simulink model "SmallSupplyChain"  (Simulink 7.9)
settings: Solver=VariableStepDiscrete  StartTime=0.0  StopTime=1000.0  RelTol=1e-3
undefined symbols (not defined in the file): des, gcbh
libraries: se_batching x2
settings Model: Creator=tsprock3  LastModifiedBy=tsprock3
settings DebuggingCC: SimStateOlderReleaseMsg=warning

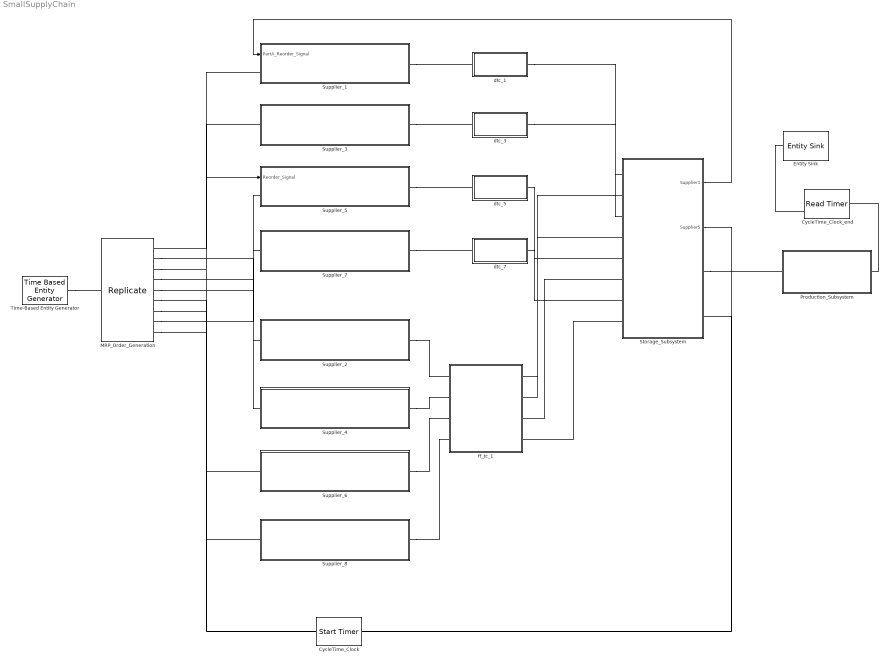
== system SmallSupplyChain ==
  CycleTime_Clock : StartTimer
  CycleTime_Clock_end : ReadTimer  TimerModeOption=Ignore  StatAverageTimeElapsed=on
      settings: OutputPortMap=o3
  Entity Sink : EntitySink
  MRP_Order_Generation : Replicate  NumberOutputPorts=9  ReplicateEntityWhen=Any entity output port is not blocked
  Production_Subsystem : Subsystem  TreatAsAtomicUnit=on
  Storage_Subsystem : Subsystem  TreatAsAtomicUnit=on
  Supplier_1 : Subsystem
  Supplier_2 : Subsystem
  Supplier_3 : Subsystem
  Supplier_4 : Subsystem
  Supplier_5 : Subsystem  mask{NumberOfServers=1, Capacity=25}
      mask prompts: NumberOfServers "Number of servers:"
  Supplier_6 : Subsystem
  Supplier_7 : Subsystem
  Supplier_8 : Subsystem
  Time-Based Entity Generator : TimeBasedEntityGenerator  Period=5
  dtc_1 : Subsystem
  dtc_3 : Subsystem
  dtc_5 : Subsystem
  dtc_7 : Subsystem
  ff_tc_1 : Subsystem  TreatAsAtomicUnit=on
  wires:
  Storage_Subsystem/1(Supplier1) -> Supplier_1/1(PartA_Reorder_Signal)
  Storage_Subsystem/2(Supplier5) -> Supplier_5/1(Reorder_Signal)
  connections:
  MRP_Order_Generation/RConn2 -- Supplier_2/LConn1
  MRP_Order_Generation/RConn4 -- Supplier_4/LConn1
  MRP_Order_Generation/RConn6 -- Supplier_6/LConn1
  MRP_Order_Generation/RConn8 -- Supplier_7/LConn1
  MRP_Order_Generation/RConn7 -- Supplier_8/LConn1
  Supplier_1/RConn1 -- dtc_1/LConn1
  Supplier_3/RConn1 -- dtc_3/LConn1
  Supplier_5/RConn1 -- dtc_5/LConn1
  Supplier_7/RConn1 -- dtc_7/LConn1
  Storage_Subsystem/RConn1 -- Production_Subsystem/LConn1
  dtc_1/RConn1 -- Storage_Subsystem/LConn1
  dtc_3/RConn1 -- Storage_Subsystem/LConn3
  dtc_5/RConn1 -- Storage_Subsystem/LConn5
  dtc_7/RConn1 -- Storage_Subsystem/LConn7
  Time-Based Entity Generator/RConn1 -- MRP_Order_Generation/LConn1
  Production_Subsystem/RConn1 -- CycleTime_Clock_end/LConn1
  CycleTime_Clock_end/RConn1 -- Entity Sink/LConn1
  MRP_Order_Generation/RConn9 -- CycleTime_Clock/LConn1
  CycleTime_Clock/RConn1 -- Storage_Subsystem/RConn2
  Supplier_1/LConn1 -- MRP_Order_Generation/RConn1
  MRP_Order_Generation/RConn3 -- Supplier_3/LConn1
  MRP_Order_Generation/RConn5 -- Supplier_5/LConn1
  Supplier_2/RConn1 -- ff_tc_1/LConn1
  Supplier_4/RConn1 -- ff_tc_1/LConn2
  Supplier_6/RConn1 -- ff_tc_1/LConn3
  Supplier_8/RConn1 -- ff_tc_1/LConn4
  Storage_Subsystem/LConn2 -- ff_tc_1/RConn2
  Storage_Subsystem/LConn4 -- ff_tc_1/RConn1
  Storage_Subsystem/LConn8 -- ff_tc_1/RConn4
  Storage_Subsystem/LConn6 -- ff_tc_1/RConn3

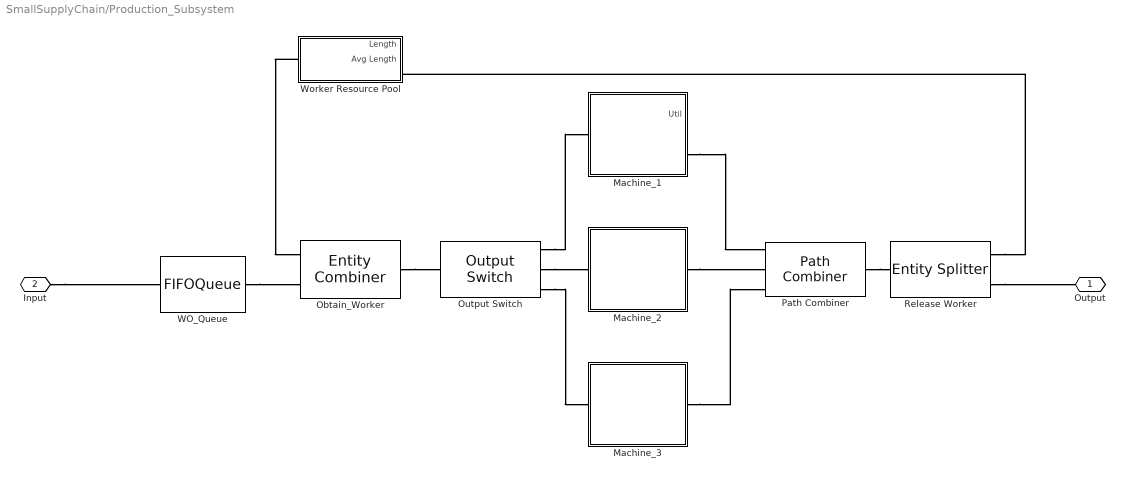
== system SmallSupplyChain/Production_Subsystem ==
  Machine_1 : Subsystem  mask{mttf=25, mttr=5, ct=3}
      mask prompts: mttf "MTTF (exp)"; mttr "MTTR (exp)"; ct "Process_Time (exp)"
  Machine_2 : Subsystem  mask{mttf=25, mttr=5, ct=3}
      mask prompts: mttf "MTTF (exp)"; mttr "MTTR (exp)"; ct "Process_Time (exp)"
  Machine_3 : Subsystem  mask{mttf=25, mttr=5, ct=3}
      mask prompts: mttf "MTTF (exp)"; mttr "MTTR (exp)"; ct "Process_Time (exp)"
  Obtain_Worker : EntityCombiner  NumberInputPorts=2
  Output Switch : OutputSwitch
  Path Combiner : PathCombiner
  Release Worker : EntitySplitter  NumberOutputPorts=2
  WO_Queue : FIFOQueue
  Worker Resource Pool : Subsystem  mask{NumberOfEventsPerPeriod=4}
      mask prompts: NumberOfEventsPerPeriod "# of Workers"
  Output : PMIOPort  Port=1  Side=Right
  Input : PMIOPort  Port=2  Side=Left
  connections:
  Input/RConn1 -- WO_Queue/LConn1
  WO_Queue/RConn1 -- Obtain_Worker/LConn2
  Worker Resource Pool/LConn1 -- Obtain_Worker/LConn1
  Obtain_Worker/RConn1 -- Output Switch/LConn1
  Output Switch/RConn1 -- Machine_1/LConn1
  Output Switch/RConn2 -- Machine_2/LConn1
  Output Switch/RConn3 -- Machine_3/LConn1
  Machine_2/RConn1 -- Path Combiner/LConn2
  Machine_1/RConn1 -- Path Combiner/LConn1
  Machine_3/RConn1 -- Path Combiner/LConn3
  Path Combiner/RConn1 -- Release Worker/LConn1
  Release Worker/RConn1 -- Worker Resource Pool/RConn1
  Release Worker/RConn2 -- Output/RConn1

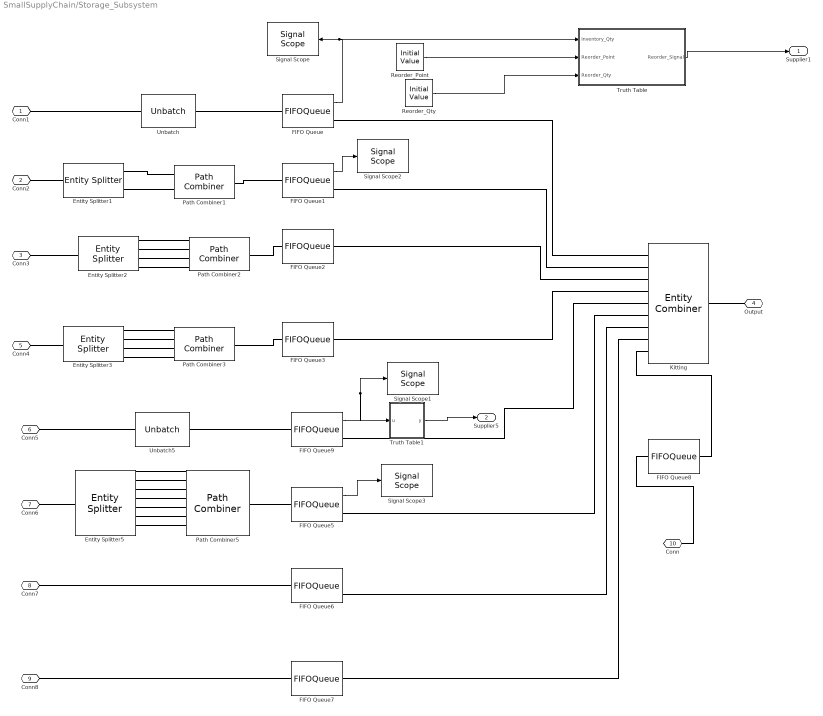
== system SmallSupplyChain/Storage_Subsystem ==
  Entity Splitter1 : EntitySplitter  NumberOutputPorts=2  ActionUponBlocking=Warn and discard entity
  Entity Splitter2 : EntitySplitter  NumberOutputPorts=4  ActionUponBlocking=Warn and discard entity
  Entity Splitter3 : EntitySplitter  NumberOutputPorts=4  ActionUponBlocking=Warn and discard entity
  Entity Splitter5 : EntitySplitter  NumberOutputPorts=8  ActionUponBlocking=Discard entity
  FIFO Queue : FIFOQueue  Capacity=100  StatNumberInBlock=on
      settings: OutputPortMap=o1
  FIFO Queue1 : FIFOQueue  Capacity=1000  StatNumberInBlock=on
      settings: OutputPortMap=o1
  FIFO Queue2 : FIFOQueue  Capacity=1000
  FIFO Queue3 : FIFOQueue  Capacity=1000
  FIFO Queue5 : FIFOQueue  Capacity=1000  StatNumberInBlock=on
      settings: OutputPortMap=o1
  FIFO Queue6 : FIFOQueue  StatNumberInBlock=on
      settings: OutputPortMap=o1
  FIFO Queue7 : FIFOQueue
  FIFO Queue8 : FIFOQueue  Capacity=inf
  FIFO Queue9 : FIFOQueue  Capacity=100  StatNumberInBlock=on
      settings: OutputPortMap=o1
  Kitting : EntityCombiner  NumberInputPorts=9  RetainComponentEntities=off
  Path Combiner1 : PathCombiner  NumberInputPorts=2
  Path Combiner2 : PathCombiner  NumberInputPorts=4
  Path Combiner3 : PathCombiner  NumberInputPorts=4
  Path Combiner5 : PathCombiner  NumberInputPorts=8
  Reorder_Point : InitialValue  InitialValue=2
  Reorder_Qty : InitialValue  InitialValue=2
  Signal Scope{,1..3} (4 alike) : SignalScope  LoadFcn=des.scope.CallbackSupport('seLoadFcn',gcbh)  StartFcn=des.scope.CallbackSupport('seStartFcn',gcbh)  StopFcn=des.scope.CallbackSupport('seStopFcn',gcbh)
      settings: CopyFcn=des.scope.CallbackSupport('seCopyFcn',gcbh)  DeleteFcn=des.scope.CallbackSupport('seDeleteFcn',gcbh)  PreSaveFcn=des.scope.CallbackSupport('sePreSaveFcn',gcbh)  NameChangeFcn=des.scope.CallbackSupport('seNameChangeFcn',gcbh)  OpenFcn=des.scope.CallbackSupport('seOpenFcn',gcbh)
  Truth Table : Truth Table  TreatAsAtomicUnit=on
  Truth Table1 : Truth Table  TreatAsAtomicUnit=on
  Unbatch : se_batching/Unbatch  Q=2
  Unbatch5 : se_batching/Unbatch  Q=8
  Conn1 : PMIOPort  Port=1  Side=Left
  Conn2 : PMIOPort  Port=2  Side=Left
  Conn3 : PMIOPort  Port=3  Side=Left
  Output : PMIOPort  Port=4  Side=Right
  Conn4 : PMIOPort  Port=5  Side=Left
  Conn5 : PMIOPort  Port=6  Side=Left
  Conn6 : PMIOPort  Port=7  Side=Left
  Conn7 : PMIOPort  Port=8  Side=Left
  Conn8 : PMIOPort  Port=9  Side=Left
  Conn : PMIOPort  Port=10  Side=Right
  Supplier1 : Outport
  Supplier5 : Outport  Port=2
  wires:
  Truth Table/1(Reorder_Signal) -> Supplier1/1
  FIFO Queue9/1 -> Signal Scope1/1, Truth Table1/1(u)
  Truth Table1/1(y) -> Supplier5/1
  FIFO Queue1/1 -> Signal Scope2/1
  FIFO Queue5/1 -> Signal Scope3/1
  Reorder_Point/1 -> Truth Table/2(Reorder_Point)
  Reorder_Qty/1 -> Truth Table/3(Reorder_Qty)
  FIFO Queue/1 -> Signal Scope/1, Truth Table/1(Inventory_Qty)
  connections:
  FIFO Queue/RConn1 -- Kitting/LConn1
  FIFO Queue1/RConn1 -- Kitting/LConn2
  FIFO Queue2/RConn1 -- Kitting/LConn3
  FIFO Queue3/RConn1 -- Kitting/LConn4
  FIFO Queue9/RConn1 -- Kitting/LConn5
  FIFO Queue5/RConn1 -- Kitting/LConn6
  FIFO Queue6/RConn1 -- Kitting/LConn7
  Kitting/LConn8 -- FIFO Queue7/RConn1
  Output/RConn1 -- Kitting/RConn1
  Conn7/RConn1 -- FIFO Queue6/LConn1
  Conn8/RConn1 -- FIFO Queue7/LConn1
  Conn2/RConn1 -- Entity Splitter1/LConn1
  Path Combiner1/RConn1 -- FIFO Queue1/LConn1
  Conn3/RConn1 -- Entity Splitter2/LConn1
  Path Combiner2/RConn1 -- FIFO Queue2/LConn1
  Conn4/RConn1 -- Entity Splitter3/LConn1
  Path Combiner3/RConn1 -- FIFO Queue3/LConn1
  Conn6/RConn1 -- Entity Splitter5/LConn1
  Path Combiner5/RConn1 -- FIFO Queue5/LConn1
  Conn/RConn1 -- FIFO Queue8/LConn1
  FIFO Queue8/RConn1 -- Kitting/LConn9
  Entity Splitter1/RConn1 -- Path Combiner1/LConn1
  Entity Splitter1/RConn2 -- Path Combiner1/LConn2
  Entity Splitter2/RConn1 -- Path Combiner2/LConn1
  Entity Splitter2/RConn2 -- Path Combiner2/LConn2
  Entity Splitter2/RConn3 -- Path Combiner2/LConn3
  Entity Splitter2/RConn4 -- Path Combiner2/LConn4
  Entity Splitter3/RConn3 -- Path Combiner3/LConn3
  Entity Splitter3/RConn4 -- Path Combiner3/LConn4
  Entity Splitter3/RConn2 -- Path Combiner3/LConn2
  Entity Splitter3/RConn1 -- Path Combiner3/LConn1
  Entity Splitter5/RConn2 -- Path Combiner5/LConn2
  Entity Splitter5/RConn3 -- Path Combiner5/LConn3
  Entity Splitter5/RConn7 -- Path Combiner5/LConn7
  Entity Splitter5/RConn5 -- Path Combiner5/LConn5
  Entity Splitter5/RConn1 -- Path Combiner5/LConn1
  Entity Splitter5/RConn4 -- Path Combiner5/LConn4
  Entity Splitter5/RConn6 -- Path Combiner5/LConn6
  Conn1/RConn1 -- Unbatch/LConn1
  Unbatch/RConn1 -- FIFO Queue/LConn1
  Conn5/RConn1 -- Unbatch5/LConn1
  Unbatch5/RConn1 -- FIFO Queue9/LConn1

== system SmallSupplyChain/Supplier_1 ==
  PartA_Reorder_Signal : Inport
  Infinite Server : InfiniteServer  ServiceTimeFrom=Attribute  AttributeName=LeadTime
  Part_A_Order_Gen : Subsystem  mask{leadtime=6, batchsize=8, disrupt=8, resolve=1}
      mask prompts: leadtime "LeadTime (exp)"; disrupt "Disruptions (MTTF)"; resolve "Resolution (MTTR)"
  Path Combiner1 : PathCombiner  NumberInputPorts=1
  Supplier_Disruption : Subsystem  mask{Mean=100, meanExp=25}
      mask prompts: Mean "MTTF"; meanExp "MTTR"
  Supplier_Waiting : FIFOQueue  Capacity=inf
  Output : PMIOPort  Port=1  Side=Right
  MRP_Signal : PMIOPort  Port=2  Side=Left
  wires:
  PartA_Reorder_Signal/1 -> Part_A_Order_Gen/1(Reorder_Signal)
  connections:
  Output/RConn1 -- Infinite Server/RConn1
  Supplier_Disruption/RConn1 -- Infinite Server/LConn1
  Path Combiner1/RConn1 -- Supplier_Waiting/LConn1
  Supplier_Waiting/RConn1 -- Supplier_Disruption/LConn1
  Part_A_Order_Gen/RConn1 -- Path Combiner1/LConn1

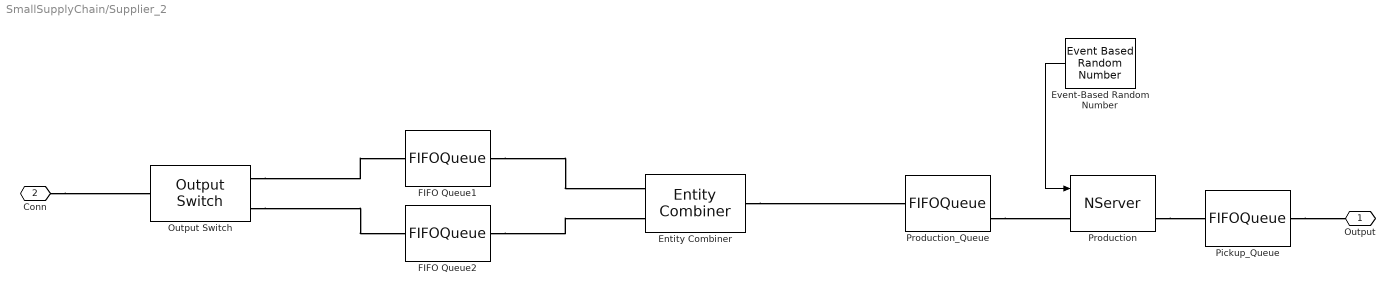
== system SmallSupplyChain/Supplier_2 ==
  Entity Combiner : EntityCombiner  NumberInputPorts=2
  Event-Based Random Number : EventBasedRandomNumber  meanExp=6  Seed=51706
  FIFO Queue1 : FIFOQueue  Capacity=1
  FIFO Queue2 : FIFOQueue  Capacity=1
  Output Switch : OutputSwitch  NumberOutputPorts=2
  Pickup_Queue : FIFOQueue
  Production : NServer  NumberOfServers=1  ServiceTimeFrom=Signal port t  StatNumberDeparted=on
  Production_Queue : FIFOQueue  StatNumberDeparted=on
  Output : PMIOPort  Port=1  Side=Right
  Conn : PMIOPort  Port=2  Side=Left
  wires:
  Event-Based Random Number/1 -> Production/1
  connections:
  Production_Queue/RConn1 -- Production/LConn1
  Output Switch/RConn1 -- FIFO Queue1/LConn1
  Output Switch/RConn2 -- FIFO Queue2/LConn1
  Conn/RConn1 -- Output Switch/LConn1
  Entity Combiner/RConn1 -- Production_Queue/LConn1
  FIFO Queue1/RConn1 -- Entity Combiner/LConn1
  FIFO Queue2/RConn1 -- Entity Combiner/LConn2
  Production/RConn1 -- Pickup_Queue/LConn1
  Pickup_Queue/RConn1 -- Output/RConn1

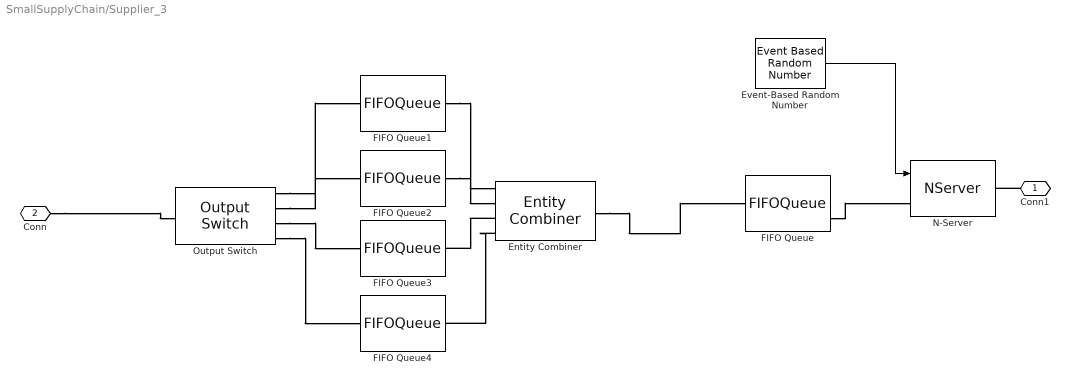
== system SmallSupplyChain/Supplier_3 ==
  Entity Combiner : EntityCombiner  NumberInputPorts=4
  Event-Based Random Number : EventBasedRandomNumber  meanExp=8  Seed=32033
  FIFO Queue : FIFOQueue  StatNumberDeparted=on
  FIFO Queue{1..4} (4 alike) : FIFOQueue  Capacity=1
  N-Server : NServer  NumberOfServers=1  ServiceTimeFrom=Signal port t
  Output Switch : OutputSwitch  NumberOutputPorts=4
  Conn1 : PMIOPort  Port=1  Side=Right
  Conn : PMIOPort  Port=2  Side=Left
  wires:
  Event-Based Random Number/1 -> N-Server/1
  connections:
  FIFO Queue/RConn1 -- N-Server/LConn1
  Conn1/RConn1 -- N-Server/RConn1
  Conn/RConn1 -- Output Switch/LConn1
  Entity Combiner/RConn1 -- FIFO Queue/LConn1
  FIFO Queue1/RConn1 -- Entity Combiner/LConn1
  Output Switch/RConn1 -- FIFO Queue1/LConn1
  FIFO Queue2/RConn1 -- Entity Combiner/LConn2
  Output Switch/RConn2 -- FIFO Queue2/LConn1
  Output Switch/RConn3 -- FIFO Queue3/LConn1
  Output Switch/RConn4 -- FIFO Queue4/LConn1
  Entity Combiner/LConn3 -- FIFO Queue3/RConn1
  Entity Combiner/LConn4 -- FIFO Queue4/RConn1

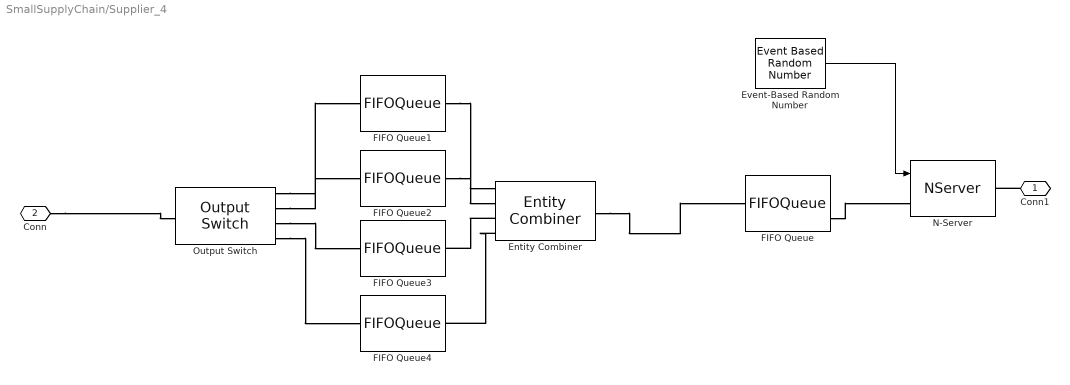
== system SmallSupplyChain/Supplier_4 ==
  Entity Combiner : EntityCombiner  NumberInputPorts=4
  Event-Based Random Number : EventBasedRandomNumber  meanExp=8  Seed=35250
  FIFO Queue : FIFOQueue  StatNumberDeparted=on
  FIFO Queue{1..4} (4 alike) : FIFOQueue  Capacity=1
  N-Server : NServer  NumberOfServers=1  ServiceTimeFrom=Signal port t
  Output Switch : OutputSwitch  NumberOutputPorts=4
  Conn1 : PMIOPort  Port=1  Side=Right
  Conn : PMIOPort  Port=2  Side=Left
  wires:
  Event-Based Random Number/1 -> N-Server/1
  connections:
  FIFO Queue/RConn1 -- N-Server/LConn1
  Conn1/RConn1 -- N-Server/RConn1
  Conn/RConn1 -- Output Switch/LConn1
  Entity Combiner/RConn1 -- FIFO Queue/LConn1
  FIFO Queue1/RConn1 -- Entity Combiner/LConn1
  Output Switch/RConn1 -- FIFO Queue1/LConn1
  FIFO Queue2/RConn1 -- Entity Combiner/LConn2
  Output Switch/RConn2 -- FIFO Queue2/LConn1
  Output Switch/RConn3 -- FIFO Queue3/LConn1
  Output Switch/RConn4 -- FIFO Queue4/LConn1
  Entity Combiner/LConn3 -- FIFO Queue3/RConn1
  Entity Combiner/LConn4 -- FIFO Queue4/RConn1

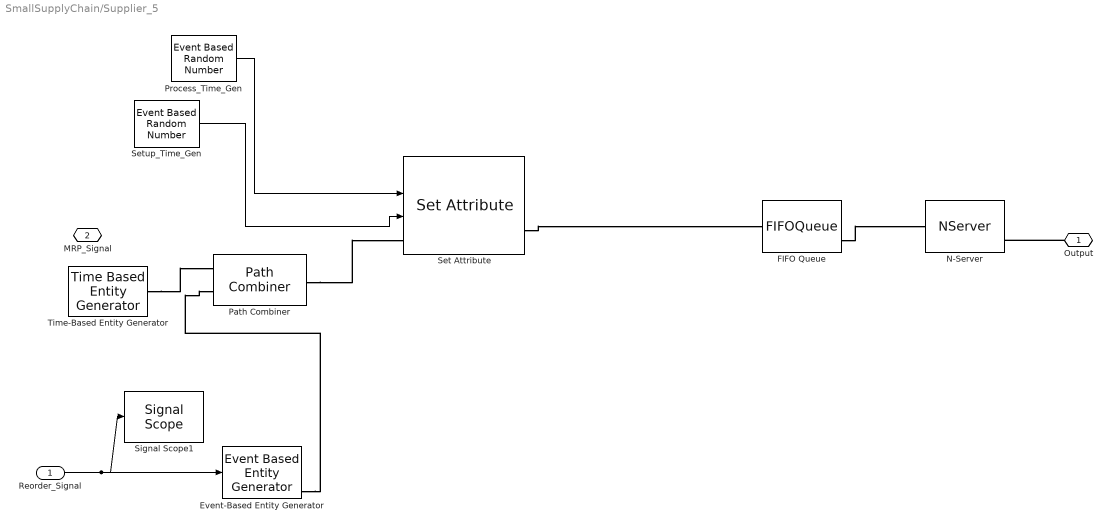
== system SmallSupplyChain/Supplier_5 ==
  Reorder_Signal : Inport
  Event-Based Entity Generator : EventBasedEntityGenerator  EntityType=Standard  StatNumberDeparted=on  StatPendingEntity=on
      settings: OutputPortMap=o0,o1
  FIFO Queue : FIFOQueue  Capacity=Capacity  StatNumberInBlock=on
      settings: OutputPortMap=o1
  N-Server : NServer  NumberOfServers=NumberOfServers  ServiceTimeFrom=Attribute  AttributeName=Process_Time  StatNumberInBlock=on
      settings: OutputPortMap=o1
  Path Combiner : PathCombiner  NumberInputPorts=2
  Process_Time_Gen : EventBasedRandomNumber  meanExp=6  Seed=17144
  Set Attribute : SetAttribute  AttributeName=Batch_Size|Process_Time|Setup_Time  AttributeFrom=Signal port|Signal port|Signal port  AttributeValue=2|1|1  AttributeTreatAsVector=1|1|1  StatNumberDeparted=on  EvaluatedAttributeValue={[];[];[]}
      settings: InputPortMap=u0,u1,u2
  Setup_Time_Gen : EventBasedRandomNumber  meanExp=0.5  Seed=24774
  Signal Scope1 : SignalScope  LoadFcn=des.scope.CallbackSupport('seLoadFcn',gcbh)  StartFcn=des.scope.CallbackSupport('seStartFcn',gcbh)  StopFcn=des.scope.CallbackSupport('seStopFcn',gcbh)
      settings: CopyFcn=des.scope.CallbackSupport('seCopyFcn',gcbh)  DeleteFcn=des.scope.CallbackSupport('seDeleteFcn',gcbh)  PreSaveFcn=des.scope.CallbackSupport('sePreSaveFcn',gcbh)  NameChangeFcn=des.scope.CallbackSupport('seNameChangeFcn',gcbh)  OpenFcn=des.scope.CallbackSupport('seOpenFcn',gcbh)
  Time-Based Entity Generator : TimeBasedEntityGenerator  Period=1000
  Output : PMIOPort  Port=1  Side=Right
  MRP_Signal : PMIOPort  Port=2  Side=Left
  wires:
  Process_Time_Gen/1 -> Set Attribute/2
  Setup_Time_Gen/1 -> Set Attribute/3
  Reorder_Signal/1 -> Signal Scope1/1, Event-Based Entity Generator/1
  connections:
  FIFO Queue/RConn1 -- N-Server/LConn1
  Output/RConn1 -- N-Server/RConn1
  Set Attribute/RConn1 -- FIFO Queue/LConn1
  Event-Based Entity Generator/RConn1 -- Path Combiner/LConn2
  Path Combiner/RConn1 -- Set Attribute/LConn1
  Time-Based Entity Generator/RConn1 -- Path Combiner/LConn1

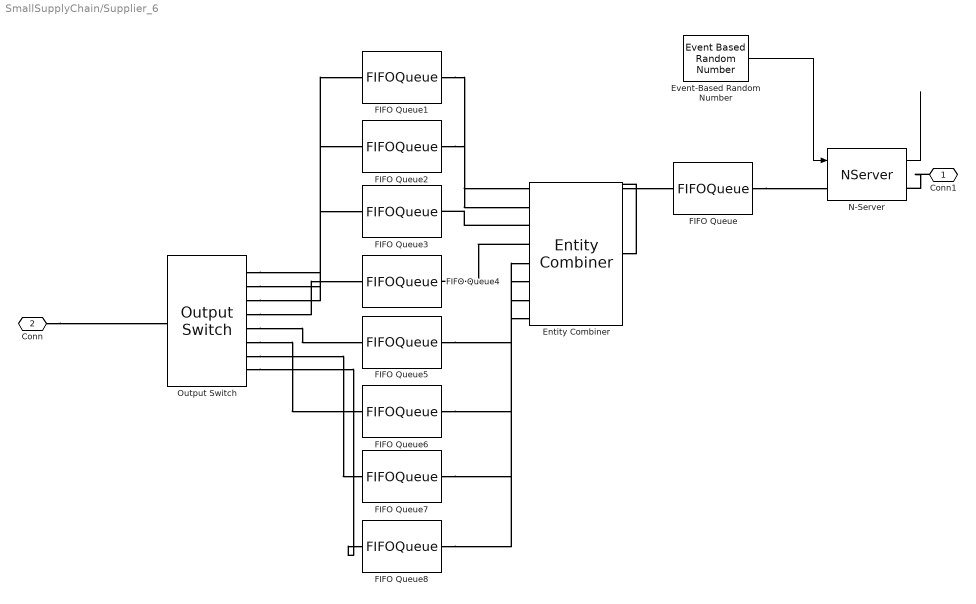
== system SmallSupplyChain/Supplier_6 ==
  Entity Combiner : EntityCombiner  NumberInputPorts=8
  Event-Based Random Number : EventBasedRandomNumber  meanExp=8  Seed=41684
  FIFO Queue : FIFOQueue
  FIFO Queue{1..8} (8 alike) : FIFOQueue  Capacity=1
  N-Server : NServer  NumberOfServers=1  ServiceTimeFrom=Signal port t  StatUtilization=on
      settings: OutputPortMap=o5
  Output Switch : OutputSwitch  NumberOutputPorts=8
  Conn1 : PMIOPort  Port=1  Side=Right
  Conn : PMIOPort  Port=2  Side=Left
  wires:
  Event-Based Random Number/1 -> N-Server/1
  N-Server/1 -> ?
  connections:
  FIFO Queue/RConn1 -- N-Server/LConn1
  Conn1/RConn1 -- N-Server/RConn1
  Conn/RConn1 -- Output Switch/LConn1
  Entity Combiner/RConn1 -- FIFO Queue/LConn1
  FIFO Queue1/RConn1 -- Entity Combiner/LConn1
  Output Switch/RConn1 -- FIFO Queue1/LConn1
  FIFO Queue2/RConn1 -- Entity Combiner/LConn2
  Output Switch/RConn2 -- FIFO Queue2/LConn1
  Output Switch/RConn3 -- FIFO Queue3/LConn1
  Output Switch/RConn4 -- FIFO Queue4/LConn1
  Entity Combiner/LConn3 -- FIFO Queue3/RConn1
  Entity Combiner/LConn4 -- FIFO Queue4/RConn1
  Output Switch/RConn5 -- FIFO Queue5/LConn1
  Output Switch/RConn6 -- FIFO Queue6/LConn1
  Output Switch/RConn7 -- FIFO Queue7/LConn1
  Output Switch/RConn8 -- FIFO Queue8/LConn1
  FIFO Queue5/RConn1 -- Entity Combiner/LConn5
  FIFO Queue6/RConn1 -- Entity Combiner/LConn6
  FIFO Queue7/RConn1 -- Entity Combiner/LConn7
  FIFO Queue8/RConn1 -- Entity Combiner/LConn8

== system SmallSupplyChain/Supplier_7 ==
  Event-Based Random Number : EventBasedRandomNumber  meanExp=5  Seed=50510
  FIFO Queue : FIFOQueue  StatAverageQueueLength=on
      settings: OutputPortMap=o3
  N-Server : NServer  ServiceTimeFrom=Signal port t
  Conn1 : PMIOPort  Port=1  Side=Right
  Conn : PMIOPort  Port=2  Side=Left
  wires:
  Event-Based Random Number/1 -> N-Server/1
  connections:
  FIFO Queue/RConn1 -- N-Server/LConn1
  Conn1/RConn1 -- N-Server/RConn1
  Conn/RConn1 -- FIFO Queue/LConn1

== system SmallSupplyChain/Supplier_8 ==
  Event-Based Random Number : EventBasedRandomNumber  Distribution=Uniform  meanExp=5  minUnif=5  maxUnif=5  Seed=53727
  FIFO Queue : FIFOQueue  StatNumberInBlock=on
      settings: OutputPortMap=o1
  N-Server : NServer  ServiceTimeFrom=Signal port t  StatUtilization=on
      settings: OutputPortMap=o5
  Signal Scope : SignalScope  LoadFcn=des.scope.CallbackSupport('seLoadFcn',gcbh)  StartFcn=des.scope.CallbackSupport('seStartFcn',gcbh)  StopFcn=des.scope.CallbackSupport('seStopFcn',gcbh)
      settings: CopyFcn=des.scope.CallbackSupport('seCopyFcn',gcbh)  DeleteFcn=des.scope.CallbackSupport('seDeleteFcn',gcbh)  PreSaveFcn=des.scope.CallbackSupport('sePreSaveFcn',gcbh)  NameChangeFcn=des.scope.CallbackSupport('seNameChangeFcn',gcbh)  OpenFcn=des.scope.CallbackSupport('seOpenFcn',gcbh)
  Signal Scope1 : SignalScope  LoadFcn=des.scope.CallbackSupport('seLoadFcn',gcbh)  StartFcn=des.scope.CallbackSupport('seStartFcn',gcbh)  StopFcn=des.scope.CallbackSupport('seStopFcn',gcbh)
      settings: CopyFcn=des.scope.CallbackSupport('seCopyFcn',gcbh)  DeleteFcn=des.scope.CallbackSupport('seDeleteFcn',gcbh)  PreSaveFcn=des.scope.CallbackSupport('sePreSaveFcn',gcbh)  NameChangeFcn=des.scope.CallbackSupport('seNameChangeFcn',gcbh)  OpenFcn=des.scope.CallbackSupport('seOpenFcn',gcbh)
  Conn1 : PMIOPort  Port=1  Side=Right
  Conn : PMIOPort  Port=2  Side=Left
  wires:
  Event-Based Random Number/1 -> N-Server/1
  N-Server/1 -> Signal Scope/1
  FIFO Queue/1 -> Signal Scope1/1
  connections:
  FIFO Queue/RConn1 -- N-Server/LConn1
  Conn1/RConn1 -- N-Server/RConn1
  Conn/RConn1 -- FIFO Queue/LConn1

== system SmallSupplyChain/dtc_1 ==
  Event-Based Random Number : EventBasedRandomNumber  Seed=56944
  Single Server : SingleServer  ServiceTimeFrom=Signal port t
  Input : PMIOPort  Port=1  Side=Left
  Output : PMIOPort  Port=2  Side=Right
  wires:
  Event-Based Random Number/1 -> Single Server/1
  connections:
  Input/RConn1 -- Single Server/LConn1
  Single Server/RConn1 -- Output/RConn1

== system SmallSupplyChain/dtc_3 ==
  Event-Based Random Number : EventBasedRandomNumber  Seed=63378
  Single Server : SingleServer  ServiceTimeFrom=Signal port t
  Conn : PMIOPort  Port=1  Side=Left
  Conn1 : PMIOPort  Port=2  Side=Right
  wires:
  Event-Based Random Number/1 -> Single Server/1
  connections:
  Conn/RConn1 -- Single Server/LConn1
  Single Server/RConn1 -- Conn1/RConn1

== system SmallSupplyChain/dtc_5 ==
  Event-Based Random Number : EventBasedRandomNumber  Seed=4276
  Single Server : SingleServer  ServiceTimeFrom=Signal port t
  Conn : PMIOPort  Port=1  Side=Left
  Conn1 : PMIOPort  Port=2  Side=Right
  wires:
  Event-Based Random Number/1 -> Single Server/1
  connections:
  Conn/RConn1 -- Single Server/LConn1
  Single Server/RConn1 -- Conn1/RConn1

== system SmallSupplyChain/dtc_7 ==
  Event-Based Random Number : EventBasedRandomNumber  Seed=10710
  Single Server : SingleServer  ServiceTimeFrom=Signal port t
  Conn : PMIOPort  Port=1  Side=Left
  Conn1 : PMIOPort  Port=2  Side=Right
  wires:
  Event-Based Random Number/1 -> Single Server/1
  connections:
  Conn/RConn1 -- Single Server/LConn1
  Single Server/RConn1 -- Conn1/RConn1

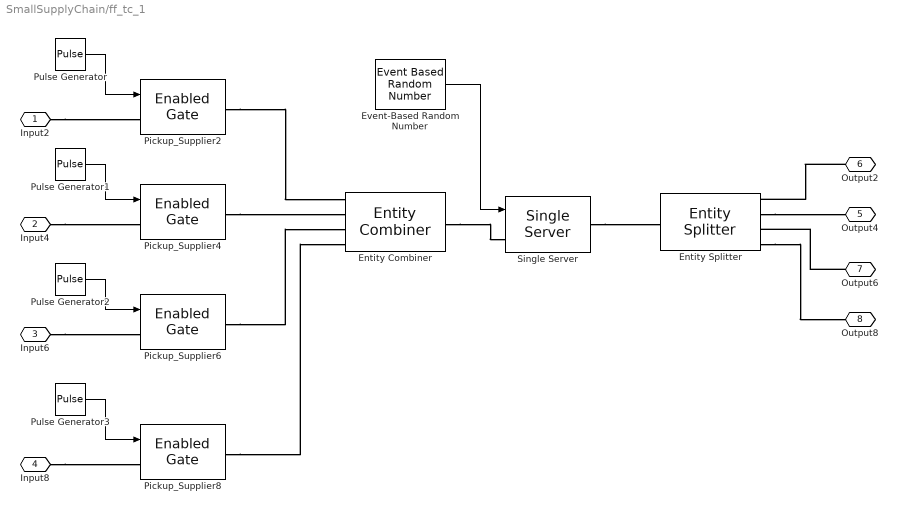
== system SmallSupplyChain/ff_tc_1 ==
  Entity Combiner : EntityCombiner  NumberInputPorts=4
  Entity Splitter : EntitySplitter  NumberOutputPorts=4  SplitEntityWhen=Any entity output port is not blocked
  Event-Based Random Number : EventBasedRandomNumber  Distribution=Uniform  meanExp=2  minUnif=1
  Pickup_Supplier{2,4,6,8} (4 alike) : EnabledGate
  Pulse Generator : DiscretePulseGenerator  PulseType=Time based  PulseWidth=5
  Pulse Generator1 : DiscretePulseGenerator  PulseType=Time based  Period=4  PulseWidth=5
  Pulse Generator2 : DiscretePulseGenerator  PulseType=Time based  Period=8  PulseWidth=5
  Pulse Generator3 : DiscretePulseGenerator  PulseType=Time based  Period=8  PulseWidth=5
  Single Server : SingleServer  ServiceTimeFrom=Signal port t
  Input2 : PMIOPort  Port=1  Side=Left
  Input4 : PMIOPort  Port=2  Side=Left
  Input6 : PMIOPort  Port=3  Side=Left
  Input8 : PMIOPort  Port=4  Side=Left
  Output4 : PMIOPort  Port=5  Side=Right
  Output2 : PMIOPort  Port=6  Side=Right
  Output6 : PMIOPort  Port=7  Side=Right
  Output8 : PMIOPort  Port=8  Side=Right
  wires:
  Pulse Generator/1 -> Pickup_Supplier2/1
  Pulse Generator1/1 -> Pickup_Supplier4/1
  Pulse Generator2/1 -> Pickup_Supplier6/1
  Pulse Generator3/1 -> Pickup_Supplier8/1
  Event-Based Random Number/1 -> Single Server/1
  connections:
  Input6/RConn1 -- Pickup_Supplier6/LConn1
  Input8/RConn1 -- Pickup_Supplier8/LConn1
  Input4/RConn1 -- Pickup_Supplier4/LConn1
  Input2/RConn1 -- Pickup_Supplier2/LConn1
  Pickup_Supplier6/RConn1 -- Entity Combiner/LConn3
  Pickup_Supplier8/RConn1 -- Entity Combiner/LConn4
  Entity Combiner/RConn1 -- Single Server/LConn1
  Single Server/RConn1 -- Entity Splitter/LConn1
  Entity Splitter/RConn2 -- Output4/RConn1
  Pickup_Supplier4/RConn1 -- Entity Combiner/LConn2
  Pickup_Supplier2/RConn1 -- Entity Combiner/LConn1
  Output2/RConn1 -- Entity Splitter/RConn1
  Output6/RConn1 -- Entity Splitter/RConn3
  Entity Splitter/RConn4 -- Output8/RConn1

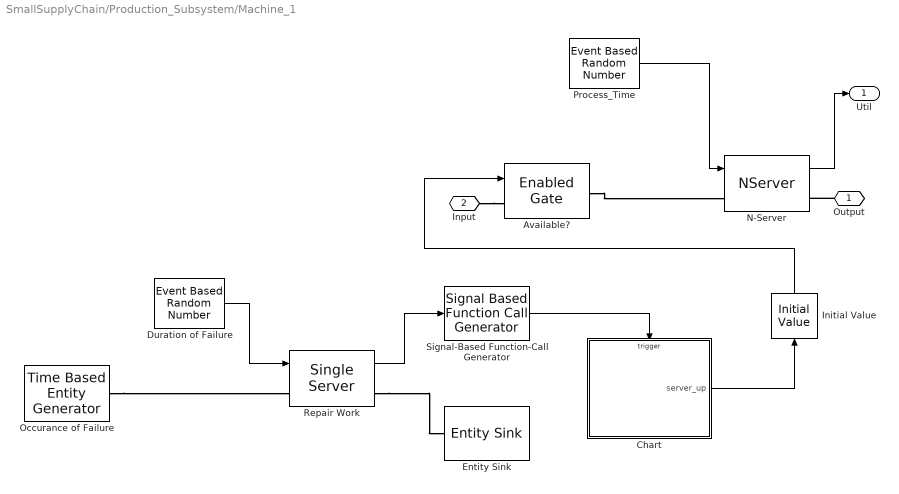
== system SmallSupplyChain/Production_Subsystem/Machine_1 ==
  Available? : EnabledGate
  Chart : Stateflow chart  TreatAsAtomicUnit=on
  Duration of Failure : EventBasedRandomNumber  meanExp=mttr  meanNorm=5  stdNorm=2
  Entity Sink : EntitySink
  Initial Value : InitialValue
  N-Server : NServer  NumberOfServers=1  ServiceTimeFrom=Signal port t  StatUtilization=on
      settings: OutputPortMap=o5
  Occurance of Failure : TimeBasedEntityGenerator  Distribution=Exponential  Mean=mttf  GenerateEntityAtSimulationStart=off  ResponseWhenUnblocked=Delayed restart
  Process_Time : EventBasedRandomNumber  meanExp=ct  Seed=27991
  Repair Work : SingleServer  ServiceTimeFrom=Signal port t  StatNumberInBlock=on
      settings: OutputPortMap=o1
  Signal-Based Function-Call Generator : SignalBasedFunctionCallGenerator  SignalEdgeOption=Either
      settings: InputPortMap=u1
  Output : PMIOPort  Port=1  Side=Right
  Input : PMIOPort  Port=2  Side=Left
  Util : Outport
  wires:
  Initial Value/1 -> Available?/1
  Chart/1(server_up) -> Initial Value/1
  Signal-Based Function-Call Generator/1 -> Chart/Trigger
  Repair Work/1 -> Signal-Based Function-Call Generator/1
  Duration of Failure/1 -> Repair Work/1
  N-Server/1 -> Util/1
  Process_Time/1 -> N-Server/1
  connections:
  Available?/RConn1 -- N-Server/LConn1
  Repair Work/RConn1 -- Entity Sink/LConn1
  Occurance of Failure/RConn1 -- Repair Work/LConn1
  Output/RConn1 -- N-Server/RConn1
  Input/RConn1 -- Available?/LConn1

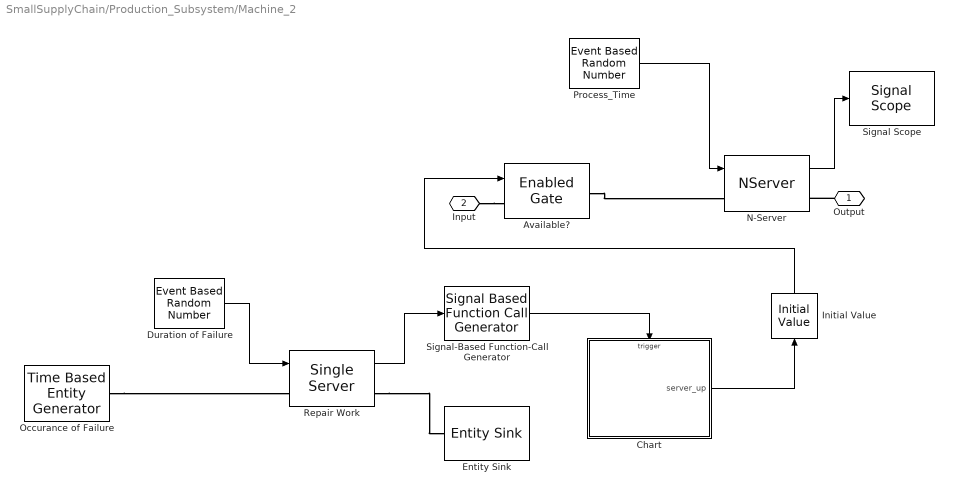
== system SmallSupplyChain/Production_Subsystem/Machine_2 ==
  Available? : EnabledGate
  Chart : Stateflow chart  TreatAsAtomicUnit=on
  Duration of Failure : EventBasedRandomNumber  meanExp=mttr  meanNorm=5  stdNorm=2
  Entity Sink : EntitySink
  Initial Value : InitialValue
  N-Server : NServer  NumberOfServers=1  ServiceTimeFrom=Signal port t  StatUtilization=on
      settings: OutputPortMap=o5
  Occurance of Failure : TimeBasedEntityGenerator  Distribution=Exponential  Mean=mttf  GenerateEntityAtSimulationStart=off  ResponseWhenUnblocked=Delayed restart
  Process_Time : EventBasedRandomNumber  meanExp=ct  Seed=27991
  Repair Work : SingleServer  ServiceTimeFrom=Signal port t  StatNumberInBlock=on
      settings: OutputPortMap=o1
  Signal Scope : SignalScope  LoadFcn=des.scope.CallbackSupport('seLoadFcn',gcbh)  StartFcn=des.scope.CallbackSupport('seStartFcn',gcbh)  StopFcn=des.scope.CallbackSupport('seStopFcn',gcbh)
      settings: CopyFcn=des.scope.CallbackSupport('seCopyFcn',gcbh)  DeleteFcn=des.scope.CallbackSupport('seDeleteFcn',gcbh)  PreSaveFcn=des.scope.CallbackSupport('sePreSaveFcn',gcbh)  NameChangeFcn=des.scope.CallbackSupport('seNameChangeFcn',gcbh)  OpenFcn=des.scope.CallbackSupport('seOpenFcn',gcbh)
  Signal-Based Function-Call Generator : SignalBasedFunctionCallGenerator  SignalEdgeOption=Either
      settings: InputPortMap=u1
  Output : PMIOPort  Port=1  Side=Right
  Input : PMIOPort  Port=2  Side=Left
  wires:
  Initial Value/1 -> Available?/1
  Chart/1(server_up) -> Initial Value/1
  Signal-Based Function-Call Generator/1 -> Chart/Trigger
  Repair Work/1 -> Signal-Based Function-Call Generator/1
  Duration of Failure/1 -> Repair Work/1
  N-Server/1 -> Signal Scope/1
  Process_Time/1 -> N-Server/1
  connections:
  Available?/RConn1 -- N-Server/LConn1
  Repair Work/RConn1 -- Entity Sink/LConn1
  Occurance of Failure/RConn1 -- Repair Work/LConn1
  Output/RConn1 -- N-Server/RConn1
  Input/RConn1 -- Available?/LConn1

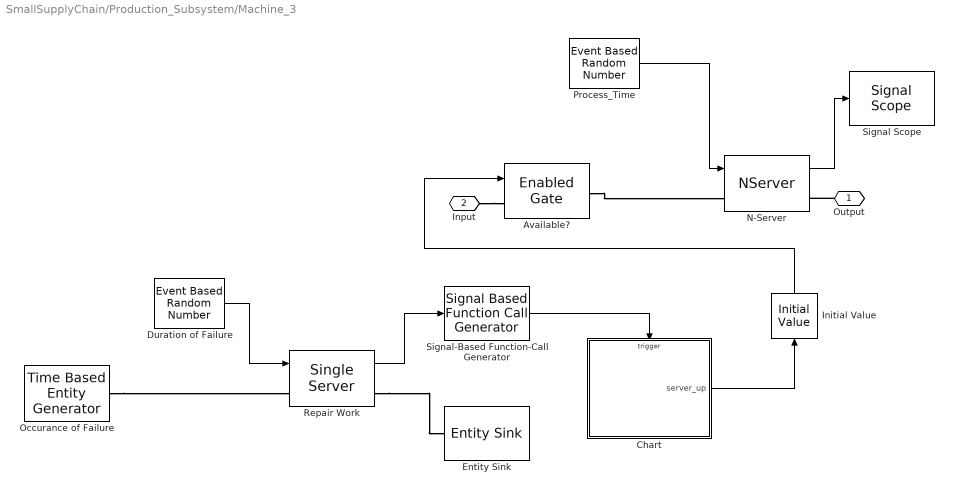
== system SmallSupplyChain/Production_Subsystem/Machine_3 ==
  Available? : EnabledGate
  Chart : Stateflow chart  TreatAsAtomicUnit=on
  Duration of Failure : EventBasedRandomNumber  meanExp=mttr  meanNorm=5  stdNorm=2
  Entity Sink : EntitySink
  Initial Value : InitialValue
  N-Server : NServer  NumberOfServers=1  ServiceTimeFrom=Signal port t  StatUtilization=on
      settings: OutputPortMap=o5
  Occurance of Failure : TimeBasedEntityGenerator  Distribution=Exponential  Mean=mttf  GenerateEntityAtSimulationStart=off  ResponseWhenUnblocked=Delayed restart
  Process_Time : EventBasedRandomNumber  meanExp=ct  Seed=27991
  Repair Work : SingleServer  ServiceTimeFrom=Signal port t  StatNumberInBlock=on
      settings: OutputPortMap=o1
  Signal Scope : SignalScope  LoadFcn=des.scope.CallbackSupport('seLoadFcn',gcbh)  StartFcn=des.scope.CallbackSupport('seStartFcn',gcbh)  StopFcn=des.scope.CallbackSupport('seStopFcn',gcbh)
      settings: CopyFcn=des.scope.CallbackSupport('seCopyFcn',gcbh)  DeleteFcn=des.scope.CallbackSupport('seDeleteFcn',gcbh)  PreSaveFcn=des.scope.CallbackSupport('sePreSaveFcn',gcbh)  NameChangeFcn=des.scope.CallbackSupport('seNameChangeFcn',gcbh)  OpenFcn=des.scope.CallbackSupport('seOpenFcn',gcbh)
  Signal-Based Function-Call Generator : SignalBasedFunctionCallGenerator  SignalEdgeOption=Either
      settings: InputPortMap=u1
  Output : PMIOPort  Port=1  Side=Right
  Input : PMIOPort  Port=2  Side=Left
  wires:
  Initial Value/1 -> Available?/1
  Chart/1(server_up) -> Initial Value/1
  Signal-Based Function-Call Generator/1 -> Chart/Trigger
  Repair Work/1 -> Signal-Based Function-Call Generator/1
  Duration of Failure/1 -> Repair Work/1
  N-Server/1 -> Signal Scope/1
  Process_Time/1 -> N-Server/1
  connections:
  Available?/RConn1 -- N-Server/LConn1
  Repair Work/RConn1 -- Entity Sink/LConn1
  Occurance of Failure/RConn1 -- Repair Work/LConn1
  Output/RConn1 -- N-Server/RConn1
  Input/RConn1 -- Available?/LConn1

== system SmallSupplyChain/Production_Subsystem/Worker Resource Pool ==
  Event-Based Entity Generator : EventBasedEntityGenerator  GenerateEntitiesUpon=Function call from port fcn
  FIFO Queue : FIFOQueue  Capacity=5  StatNumberInBlock=on  StatAverageQueueLength=on
      settings: OutputPortMap=o1,o3
  Path Combiner : PathCombiner  NumberInputPorts=2
  Time-Based Function-Call Generator : TimeBasedFunctionCallGenerator  EventGenerationMode=Only at simulation start  NumberOfEventsPerPeriod=NumberOfEventsPerPeriod
  Return : PMIOPort  Port=1  Side=Right
  Acquire : PMIOPort  Port=2  Side=Left
  Length : Outport
  Avg Length : Outport  Port=2
  wires:
  Time-Based Function-Call Generator/1 -> Event-Based Entity Generator/1
  FIFO Queue/2 -> Avg Length/1
  FIFO Queue/1 -> Length/1
  connections:
  Event-Based Entity Generator/RConn1 -- Path Combiner/LConn1
  Path Combiner/RConn1 -- FIFO Queue/LConn1
  Return/RConn1 -- Path Combiner/LConn2
  Acquire/RConn1 -- FIFO Queue/RConn1

== system SmallSupplyChain/Supplier_1/Part_A_Order_Gen ==
  Reorder_Signal : Inport
  Batch_Size : EventBasedRandomNumber  Distribution=Uniform  meanExp=leadtime  minUnif=batchsize  maxUnif=batchsize  Seed=17144
  Event-Based Entity Generator : EventBasedEntityGenerator  EntityType=Standard
  LeadTime_Gen : EventBasedRandomNumber  meanExp=leadtime  minUnif=5  maxUnif=5  Seed=17144
  Part_Disruption : Subsystem  mask{Mean=disrupt, meanExp=resolve}
      mask prompts: Mean "MTTF"; meanExp "MTTR"
  Part_Waiting : FIFOQueue
  Path Combiner : PathCombiner  NumberInputPorts=2
  Set Attribute : SetAttribute  AttributeName=LeadTime|Batch_Size  AttributeFrom=Signal port|Signal port  AttributeValue=1|1  AttributeTreatAsVector=1|1  EvaluatedAttributeValue={[];[]}
      settings: InputPortMap=u0,u1
  Time-Based Entity Generator : TimeBasedEntityGenerator  Period=1000
  WO_Ready : PMIOPort  Port=1  Side=Right
  wires:
  LeadTime_Gen/1 -> Set Attribute/1
  Batch_Size/1 -> Set Attribute/2
  Reorder_Signal/1 -> Event-Based Entity Generator/1
  connections:
  Event-Based Entity Generator/RConn1 -- Path Combiner/LConn2
  Part_Waiting/RConn1 -- Part_Disruption/LConn1
  Set Attribute/RConn1 -- Part_Waiting/LConn1
  Time-Based Entity Generator/RConn1 -- Path Combiner/LConn1
  Path Combiner/RConn1 -- Set Attribute/LConn1
  WO_Ready/RConn1 -- Part_Disruption/RConn1

== system SmallSupplyChain/Supplier_1/Supplier_Disruption ==
  Available? : EnabledGate
  Chart : Stateflow chart  TreatAsAtomicUnit=on
  Duration of Failure : EventBasedRandomNumber  meanExp=meanExp  meanNorm=5  stdNorm=2
  Entity Sink : EntitySink
  Initial Value : InitialValue
  Occurance of Failure : TimeBasedEntityGenerator  Distribution=Exponential  Mean=Mean  GenerateEntityAtSimulationStart=off  ResponseWhenUnblocked=Delayed restart
  Repair Work : SingleServer  ServiceTimeFrom=Signal port t  StatNumberInBlock=on
      settings: OutputPortMap=o1
  Signal-Based Function-Call Generator : SignalBasedFunctionCallGenerator  SignalEdgeOption=Either
      settings: InputPortMap=u1
  Output : PMIOPort  Port=1  Side=Right
  Input : PMIOPort  Port=2  Side=Left
  wires:
  Initial Value/1 -> Available?/1
  Chart/1(server_up) -> Initial Value/1
  Signal-Based Function-Call Generator/1 -> Chart/Trigger
  Repair Work/1 -> Signal-Based Function-Call Generator/1
  Duration of Failure/1 -> Repair Work/1
  connections:
  Repair Work/RConn1 -- Entity Sink/LConn1
  Occurance of Failure/RConn1 -- Repair Work/LConn1
  Output/RConn1 -- Available?/RConn1
  Input/RConn1 -- Available?/LConn1

== system SmallSupplyChain/Supplier_1/Part_A_Order_Gen/Part_Disruption ==
  Available? : EnabledGate
  Chart : Stateflow chart  TreatAsAtomicUnit=on
  Duration of Failure : EventBasedRandomNumber  meanExp=meanExp  meanNorm=5  stdNorm=2
  Entity Sink : EntitySink
  Initial Value : InitialValue
  Occurance of Failure : TimeBasedEntityGenerator  Distribution=Exponential  Mean=Mean  GenerateEntityAtSimulationStart=off  ResponseWhenUnblocked=Delayed restart
  Repair Work : SingleServer  ServiceTimeFrom=Signal port t  StatNumberInBlock=on
      settings: OutputPortMap=o1
  Signal-Based Function-Call Generator : SignalBasedFunctionCallGenerator  SignalEdgeOption=Either
      settings: InputPortMap=u1
  Output : PMIOPort  Port=1  Side=Right
  Input : PMIOPort  Port=2  Side=Left
  wires:
  Initial Value/1 -> Available?/1
  Chart/1(server_up) -> Initial Value/1
  Signal-Based Function-Call Generator/1 -> Chart/Trigger
  Repair Work/1 -> Signal-Based Function-Call Generator/1
  Duration of Failure/1 -> Repair Work/1
  connections:
  Repair Work/RConn1 -- Entity Sink/LConn1
  Occurance of Failure/RConn1 -- Repair Work/LConn1
  Output/RConn1 -- Available?/RConn1
  Input/RConn1 -- Available?/LConn1

== matlab function Storage_Subsystem/Truth Table1 ==
  data: u input double; y output double
function y = fcn(u)

aVarTruthTableCondition_1 = false;


% Reorder

aVarTruthTableCondition_1 = logical(u == 8);

if (aVarTruthTableCondition_1)
    aFcnTruthTableAction_1();
else % Default
    aFcnTruthTableAction_2();
end

function aFcnTruthTableAction_1()

% Reorder

y = 1;

function aFcnTruthTableAction_2()

% Wait

y = 0;

== matlab function Storage_Subsystem/Truth Table ==
  data: Inventory_Qty input double; Reorder_Signal output double; Reorder_Point input double; Reorder_Qty input double
function Reorder_Signal = fcn(Inventory_Qty, Reorder_Point, Reorder_Qty)

aVarTruthTableCondition_1 = false;


% Reorder

aVarTruthTableCondition_1 = logical(Inventory_Qty == Reorder_Point);

if (aVarTruthTableCondition_1)
    aFcnTruthTableAction_1();
else % Default
    aFcnTruthTableAction_2();
end

function aFcnTruthTableAction_1()

% Reorder

Reorder_Signal = Reorder_Qty;

function aFcnTruthTableAction_2()

% Wait

Reorder_Signal = 0;

== stateflow chart Production_Subsystem/Machine_1/Chart ==
  state Down
    en: server_up = 0;
  state Up
    en: server_up = 1;
  (default) -> Down
  Down -> Up : event
  Up -> Down : event
  data: server_up output double
  events: event input FUNCTION_CALL_EVENT

== stateflow chart Production_Subsystem/Machine_2/Chart ==
  state Down
    en: server_up = 0;
  state Up
    en: server_up = 1;
  (default) -> Down
  Down -> Up : event
  Up -> Down : event
  data: server_up output double
  events: event input FUNCTION_CALL_EVENT

== stateflow chart Production_Subsystem/Machine_3/Chart ==
  state Down
    en: server_up = 0;
  state Up
    en: server_up = 1;
  (default) -> Down
  Down -> Up : event
  Up -> Down : event
  data: server_up output double
  events: event input FUNCTION_CALL_EVENT

== stateflow chart Supplier_1/Part_A_Order_Gen/Part_Disruption/Chart ==
  state Down
    en: server_up = 0;
  state Up
    en: server_up = 1;
  (default) -> Down
  Down -> Up : event
  Up -> Down : event
  data: server_up output double
  events: event input FUNCTION_CALL_EVENT

== stateflow chart Supplier_1/Supplier_Disruption/Chart ==
  state Down
    en: server_up = 0;
  state Up
    en: server_up = 1;
  (default) -> Down
  Down -> Up : event
  Up -> Down : event
  data: server_up output double
  events: event input FUNCTION_CALL_EVENT
